simulink model "week3_problem2_2005052"  (R2021a)
settings: Solver=VariableStepAuto  StartTime=0.0  StopTime=10.0  RelTol=1e-3
settings Model: Creator=admin  LastModifiedBy=admin
settings SolverCC: AlgebraicLoopSolver=TrustRegion
settings DebuggingCC: SFMachineParentedDataDiag=warning

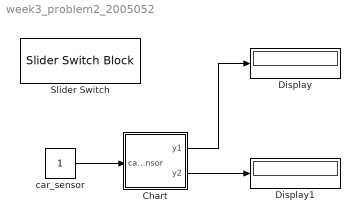
== system week3_problem2_2005052 ==
  Chart : Stateflow chart  TreatAsAtomicUnit=on
  Display : Display
  Display1 : Display
  Slider Switch : SliderSwitchBlock  LabelPosition=Hide
      settings: Values={{'Off', 'On'}, [0 1]}
  car_sensor : Constant
  wires:
  Chart/2(y2) -> Display1/1
  Chart/1(y1) -> Display/1
  car_sensor/1 -> Chart/1(car_sensor)

== stateflow chart week3_problem2_2005052/Chart ==
  state Stop
    en:y1=red;
    y2=green;
  state StopForTraffic
    en:
    y1=red;
    y2=green;
  state StopToGo
    en:
    y1=red;
    y2=yellow;
  state GoToStop
    en:
    y1=yellow;
    y2=red;
  state Go
    en:
    y1=green;
    y2=red;
  (default) -> Stop
  Stop -> StopForTraffic : after(20,sec)
  StopForTraffic -> StopToGo : [car_sensor]
  GoToStop -> Stop : after(3,sec)
  StopToGo -> Go : after(3,sec)
  Go -> GoToStop : after(10,sec)
  data: green constant double =3; yellow constant double =2; red constant double =1; y1 output; car_sensor input; y2 output
